simulink model "state_space"  (R2020b)
settings: Solver=VariableStepAuto  StartTime=0.0  StopTime=100  RelTol=1e-3
values from neighbouring files (symbols this model uses):
  A = [0 1 0 0 0; 0 0 0 0 0; 0 0 0 1 0; 0 0 0 0 1; 0 0 0 0 0]    [Kalman_vel_est.m]    (also in continues_time_state_space.m = [0 1 0 0; 0 0 0 0; 0 0 0 omega; 0 0 -omega 0])
  acc = test.data(:,28)    [acc_analysis.m]    (also in continues_time_state_space.m = 0)
  H = 100    [continues_time_state_space.m]
libraries: sharedTrackingLibrary x9, simulink x1
settings Model: Creator=Bruger  LastModifiedBy=Bruger

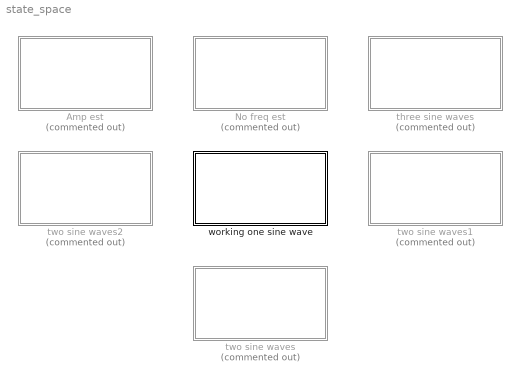
== system state_space ==
  Amp est : Subsystem  Commented=on
  No freq est : Subsystem  Commented=on
  three sine waves : Subsystem  Commented=on
  two sine waves : Subsystem  Commented=on
  two sine waves1 : Subsystem  Commented=on
  two sine waves2 : Subsystem  Commented=on
  working one sine wave : Subsystem

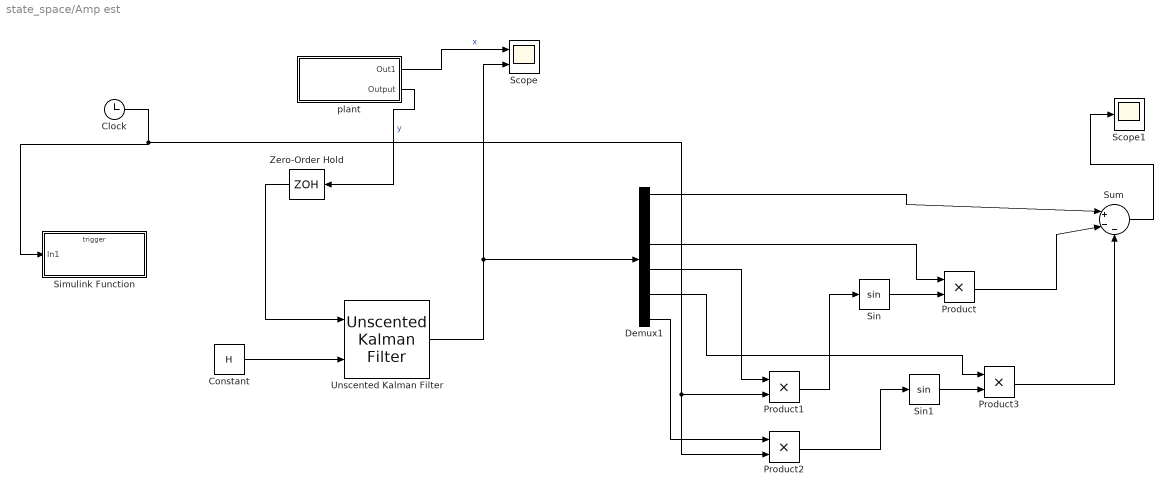
== system state_space/Amp est ==
  Clock : Clock
  Constant : Constant  Value=H
  Demux1 : Demux  Outputs=6
  Product{,1..3} (4 alike) : Product
  Scope : Scope  NumInputPorts=2
  Scope1 : Scope
  Simulink Function : Subsystem  TreatAsAtomicUnit=on
  Sin : Trigonometry
  Sin1 : Trigonometry
  Sum : Sum  Inputs=|+--
  Unscented Kalman Filter : sharedTrackingLibrary/Unscented Kalman Filter  StateTransitionFcn=state_transfer  HasAdditiveProcessNoise=Additive  ProcessNoise=0.01  HasTimeVaryingProcessNoise=off  HasStateTransitionFcnExtraArgument=0  InitialState=[100 0 40 2 20 1]  InitialStateCovariance=0.1  Alpha=1e-3  Beta=2  Kappa=0  MeasurementFcn1=f  HasMeasurementEnablePort1=off  HasAdditiveMeasurementNoise1=Additive  MeasurementNoise1=0.01  HasTimeVaryingMeasurementNoise1=off  HasMeasurementFcnExtraArgument1=0  MeasurementFcn2=measure_alt  HasMeasurementEnablePort2=off  HasAdditiveMeasurementNoise2=Additive  MeasurementNoise2=0.01  HasTimeVaryingMeasurementNoise2=off  HasMeasurementFcnExtraArgument2=0  MeasurementFcn3=myMeasurementFcn  HasMeasurementEnablePort3=off  HasAdditiveMeasurementNoise3=Additive  MeasurementNoise3=1  HasTimeVaryingMeasurementNoise3=off  HasMeasurementFcnExtraArgument3=0  MeasurementFcn4=myMeasurementFcn  HasMeasurementEnablePort4=off  HasAdditiveMeasurementNoise4=Additive  MeasurementNoise4=1  HasTimeVaryingMeasurementNoise4=off  HasMeasurementFcnExtraArgument4=0  MeasurementFcn5=myMeasurementFcn  HasMeasurementEnablePort5=off  HasAdditiveMeasurementNoise5=Additive  MeasurementNoise5=1  HasTimeVaryingMeasurementNoise5=off  HasMeasurementFcnExtraArgument5=0  EnableMultirate=off  StateTransitionFcnSampleTime=1  MeasurementFcn1SampleTime=1  MeasurementFcn2SampleTime=1  MeasurementFcn3SampleTime=1  MeasurementFcn4SampleTime=1  MeasurementFcn5SampleTime=1  UseCurrentEstimator=on  OutputStateCovariance=off  DataType=double  SampleTime=0.1  NumberOfMeasurements=2
      settings: SourceProductBaseCode=CT,DR,TF,ID,LP,NV,AR,RO,RR,UV,VE
  Zero-Order Hold : ZeroOrderHold  SampleTime=0.1
  plant : Subsystem
  wires:
  Zero-Order Hold/1 -> Unscented Kalman Filter/1
  plant/2(Output) -> Zero-Order Hold/1  "y"
  plant/1(Out1) -> Scope/1  "x"
  Constant/1 -> Unscented Kalman Filter/2
  Demux1/5 -> Product3/1
  Demux1/1 -> Sum/1
  Product3/1 -> Sum/3
  Demux1/3 -> Product/1
  Demux1/4 -> Product1/1
  Clock/1 -> Product2/2, Product1/2, Simulink Function/1(In1)
  Sin1/1 -> Product3/2
  Demux1/6 -> Product2/1
  Unscented Kalman Filter/1 -> Scope/2, Demux1/1
  Product/1 -> Sum/2
  Sin/1 -> Product/2
  Product2/1 -> Sin1/1
  Product1/1 -> Sin/1
  Sum/1 -> Scope1/1

== system state_space/No freq est ==
  Constant : Constant  Value=H
  Scope : Scope  NumInputPorts=2
  Scope1 : Scope
  Unscented Kalman Filter : sharedTrackingLibrary/Unscented Kalman Filter  StateTransitionFcn=state_transfer  HasAdditiveProcessNoise=Additive  ProcessNoise=1  HasTimeVaryingProcessNoise=off  HasStateTransitionFcnExtraArgument=0  InitialState=[100 0 0 10]  InitialStateCovariance=1  Alpha=1e-3  Beta=2  Kappa=0  MeasurementFcn1=measurement_func  HasMeasurementEnablePort1=off  HasAdditiveMeasurementNoise1=Additive  MeasurementNoise1=1  HasTimeVaryingMeasurementNoise1=off  HasMeasurementFcnExtraArgument1=0  MeasurementFcn2=measure_alt  HasMeasurementEnablePort2=off  HasAdditiveMeasurementNoise2=Additive  MeasurementNoise2=1  HasTimeVaryingMeasurementNoise2=off  HasMeasurementFcnExtraArgument2=0  MeasurementFcn3=myMeasurementFcn  HasMeasurementEnablePort3=off  HasAdditiveMeasurementNoise3=Additive  MeasurementNoise3=1  HasTimeVaryingMeasurementNoise3=off  HasMeasurementFcnExtraArgument3=0  MeasurementFcn4=myMeasurementFcn  HasMeasurementEnablePort4=off  HasAdditiveMeasurementNoise4=Additive  MeasurementNoise4=1  HasTimeVaryingMeasurementNoise4=off  HasMeasurementFcnExtraArgument4=0  MeasurementFcn5=myMeasurementFcn  HasMeasurementEnablePort5=off  HasAdditiveMeasurementNoise5=Additive  MeasurementNoise5=1  HasTimeVaryingMeasurementNoise5=off  HasMeasurementFcnExtraArgument5=0  EnableMultirate=off  StateTransitionFcnSampleTime=1  MeasurementFcn1SampleTime=1  MeasurementFcn2SampleTime=1  MeasurementFcn3SampleTime=1  MeasurementFcn4SampleTime=1  MeasurementFcn5SampleTime=1  UseCurrentEstimator=on  OutputStateCovariance=off  DataType=double  SampleTime=0.1  NumberOfMeasurements=2
      settings: SourceProductBaseCode=CT,DR,TF,ID,LP,NV,AR,RO,RR,UV,VE
  Zero-Order Hold : ZeroOrderHold  SampleTime=0.1
  plant : Subsystem
  wires:
  Zero-Order Hold/1 -> Unscented Kalman Filter/1
  plant/2(Output) -> Zero-Order Hold/1  "y"
  Unscented Kalman Filter/1 -> Scope/2
  plant/1(Out1) -> Scope/1  "x"
  Constant/1 -> Unscented Kalman Filter/2

== system state_space/three sine waves ==
  Constant : Constant  Value=H
  Demux : Demux  Outputs=11
  Demux1 : Demux  Outputs=8
  Scope : Scope  NumInputPorts=2
  Scope1 : Scope  NumInputPorts=6
  Scope2 : Scope  NumInputPorts=3
  Unscented Kalman Filter : sharedTrackingLibrary/Unscented Kalman Filter  StateTransitionFcn=state_transfer  HasAdditiveProcessNoise=Additive  ProcessNoise=1e-10  HasTimeVaryingProcessNoise=off  HasStateTransitionFcnExtraArgument=0  InitialState=[50 0 0 10 1 0 5 4 0 20 2]  InitialStateCovariance=1e-10  Alpha=1e-3  Beta=1  Kappa=0  MeasurementFcn1=measurement_func  HasMeasurementEnablePort1=off  HasAdditiveMeasurementNoise1=Additive  MeasurementNoise1=1e-10  HasTimeVaryingMeasurementNoise1=off  HasMeasurementFcnExtraArgument1=0  MeasurementFcn2=measure_alt  HasMeasurementEnablePort2=off  HasAdditiveMeasurementNoise2=Additive  MeasurementNoise2=1e-10  HasTimeVaryingMeasurementNoise2=off  HasMeasurementFcnExtraArgument2=0  MeasurementFcn3=myMeasurementFcn  HasMeasurementEnablePort3=off  HasAdditiveMeasurementNoise3=Additive  MeasurementNoise3=1  HasTimeVaryingMeasurementNoise3=off  HasMeasurementFcnExtraArgument3=0  MeasurementFcn4=myMeasurementFcn  HasMeasurementEnablePort4=off  HasAdditiveMeasurementNoise4=Additive  MeasurementNoise4=1  HasTimeVaryingMeasurementNoise4=off  HasMeasurementFcnExtraArgument4=0  MeasurementFcn5=myMeasurementFcn  HasMeasurementEnablePort5=off  HasAdditiveMeasurementNoise5=Additive  MeasurementNoise5=1  HasTimeVaryingMeasurementNoise5=off  HasMeasurementFcnExtraArgument5=0  EnableMultirate=off  StateTransitionFcnSampleTime=1  MeasurementFcn1SampleTime=1  MeasurementFcn2SampleTime=1  MeasurementFcn3SampleTime=1  MeasurementFcn4SampleTime=1  MeasurementFcn5SampleTime=1  UseCurrentEstimator=on  OutputStateCovariance=off  DataType=double  SampleTime=0.1  NumberOfMeasurements=2
      settings: SourceProductBaseCode=CT,DR,TF,ID,LP,NV,AR,RO,RR,UV,VE
  Zero-Order Hold : ZeroOrderHold  SampleTime=0.1
  plant : Subsystem
  wires:
  Zero-Order Hold/1 -> Unscented Kalman Filter/1
  plant/2(Output) -> Zero-Order Hold/1  "y"
  Unscented Kalman Filter/1 -> Scope/2, Demux/1
  plant/1(Out1) -> Demux1/1, Scope/1  "x"
  Constant/1 -> Unscented Kalman Filter/2
  Demux/6 -> Scope1/5  "sine_est2"
  Demux1/5 -> Scope1/1  "sine_gt2"
  Demux/3 -> Scope1/4  "sine_est1"
  Demux1/3 -> Scope1/2  "sine_gt1"
  Demux/8 -> Scope2/3  "freq"
  Demux/5 -> Scope2/2
  Demux/11 -> Scope2/1
  Demux1/7 -> Scope1/3  "sine_gt3"
  Demux/9 -> Scope1/6  "sine_est3"

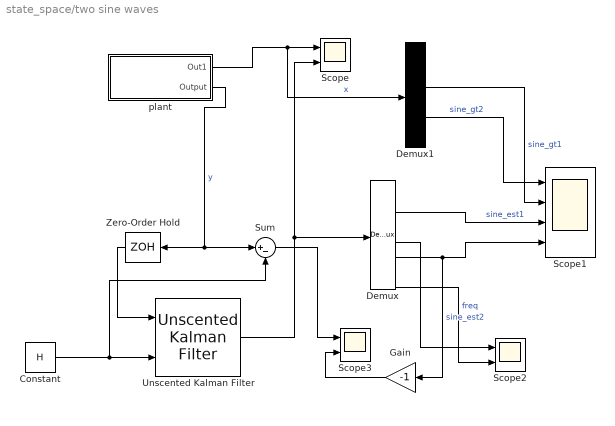
== system state_space/two sine waves ==
  Constant : Constant  Value=H
  Demux : Demux  Outputs=8
  Demux1 : Demux  Outputs=6
  Gain : Gain  Gain=-1
  Scope : Scope  NumInputPorts=2
  Scope1 : Scope  NumInputPorts=4
  Scope2 : Scope  NumInputPorts=2
  Scope3 : Scope  NumInputPorts=2
  Sum : Sum  Inputs=|+-
  Unscented Kalman Filter : sharedTrackingLibrary/Unscented Kalman Filter  StateTransitionFcn=state_transfer  HasAdditiveProcessNoise=Additive  ProcessNoise=0.1  HasTimeVaryingProcessNoise=off  HasStateTransitionFcnExtraArgument=0  InitialState=[100 0 0 40 2.5 0 20 1.5]  InitialStateCovariance=1  Alpha=1e-3  Beta=2  Kappa=0  MeasurementFcn1=measurement_func  HasMeasurementEnablePort1=off  HasAdditiveMeasurementNoise1=Additive  MeasurementNoise1=0.1  HasTimeVaryingMeasurementNoise1=off  HasMeasurementFcnExtraArgument1=0  MeasurementFcn2=measure_alt  HasMeasurementEnablePort2=off  HasAdditiveMeasurementNoise2=Additive  MeasurementNoise2=0.1  HasTimeVaryingMeasurementNoise2=off  HasMeasurementFcnExtraArgument2=0  MeasurementFcn3=myMeasurementFcn  HasMeasurementEnablePort3=off  HasAdditiveMeasurementNoise3=Additive  MeasurementNoise3=1  HasTimeVaryingMeasurementNoise3=off  HasMeasurementFcnExtraArgument3=0  MeasurementFcn4=myMeasurementFcn  HasMeasurementEnablePort4=off  HasAdditiveMeasurementNoise4=Additive  MeasurementNoise4=1  HasTimeVaryingMeasurementNoise4=off  HasMeasurementFcnExtraArgument4=0  MeasurementFcn5=myMeasurementFcn  HasMeasurementEnablePort5=off  HasAdditiveMeasurementNoise5=Additive  MeasurementNoise5=1  HasTimeVaryingMeasurementNoise5=off  HasMeasurementFcnExtraArgument5=0  EnableMultirate=off  StateTransitionFcnSampleTime=1  MeasurementFcn1SampleTime=1  MeasurementFcn2SampleTime=1  MeasurementFcn3SampleTime=1  MeasurementFcn4SampleTime=1  MeasurementFcn5SampleTime=1  UseCurrentEstimator=on  OutputStateCovariance=off  DataType=double  SampleTime=0.1  NumberOfMeasurements=2
      settings: SourceProductBaseCode=CT,DR,TF,ID,LP,NV,AR,RO,RR,UV,VE
  Zero-Order Hold : ZeroOrderHold  SampleTime=0.1
  plant : Subsystem
  wires:
  Zero-Order Hold/1 -> Unscented Kalman Filter/1
  plant/2(Output) -> Zero-Order Hold/1, Sum/1  "y"
  Unscented Kalman Filter/1 -> Scope/2, Demux/1
  plant/1(Out1) -> Demux1/1, Scope/1  "x"
  Constant/1 -> Sum/2, Unscented Kalman Filter/2
  Demux/6 -> Gain/1, Scope1/4  "sine_est2"
  Demux1/5 -> Scope1/1  "sine_gt2"
  Demux/3 -> Scope1/3  "sine_est1"
  Demux1/3 -> Scope1/2  "sine_gt1"
  Demux/8 -> Scope2/2  "freq"
  Demux/5 -> Scope2/1
  Sum/1 -> Scope3/1
  Gain/1 -> Scope3/2

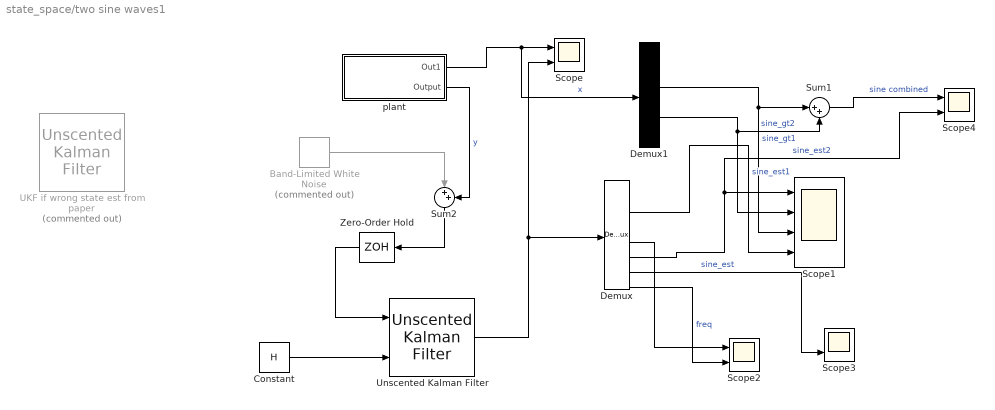
== system state_space/two sine waves1 ==
  Band-Limited White Noise : simulink/Sources/Band-Limited White Noise  Commented=on  Cov=[0.1]  Ts=0.05  seed=[23341]
  Constant : Constant  Value=H
  Demux : Demux  Outputs=8
  Demux1 : Demux  Outputs=6
  Scope{,2..4} (4 alike) : Scope  NumInputPorts=2
  Scope1 : Scope  NumInputPorts=4
  Sum1 : Sum  Inputs=|++
  Sum2 : Sum  Inputs=|++
  UKF if wrong state est from paper : sharedTrackingLibrary/Unscented Kalman Filter  Commented=on  StateTransitionFcn=state_transfer  HasAdditiveProcessNoise=Additive  ProcessNoise=0.01  HasTimeVaryingProcessNoise=off  HasStateTransitionFcnExtraArgument=0  InitialState=[100 0 0 20 0.5 0 40 1]  InitialStateCovariance=0.01  Alpha=1e-3  Beta=2  Kappa=0  MeasurementFcn1=measurement_func  HasMeasurementEnablePort1=off  HasAdditiveMeasurementNoise1=Additive  MeasurementNoise1=0.04  HasTimeVaryingMeasurementNoise1=off  HasMeasurementFcnExtraArgument1=0  MeasurementFcn2=measure_alt  HasMeasurementEnablePort2=off  HasAdditiveMeasurementNoise2=Additive  MeasurementNoise2=0.1  HasTimeVaryingMeasurementNoise2=off  HasMeasurementFcnExtraArgument2=0  MeasurementFcn3=myMeasurementFcn  HasMeasurementEnablePort3=off  HasAdditiveMeasurementNoise3=Additive  MeasurementNoise3=1  HasTimeVaryingMeasurementNoise3=off  HasMeasurementFcnExtraArgument3=0  MeasurementFcn4=myMeasurementFcn  HasMeasurementEnablePort4=off  HasAdditiveMeasurementNoise4=Additive  MeasurementNoise4=1  HasTimeVaryingMeasurementNoise4=off  HasMeasurementFcnExtraArgument4=0  MeasurementFcn5=myMeasurementFcn  HasMeasurementEnablePort5=off  HasAdditiveMeasurementNoise5=Additive  MeasurementNoise5=1  HasTimeVaryingMeasurementNoise5=off  HasMeasurementFcnExtraArgument5=0  EnableMultirate=off  StateTransitionFcnSampleTime=1  MeasurementFcn1SampleTime=1  MeasurementFcn2SampleTime=1  MeasurementFcn3SampleTime=1  MeasurementFcn4SampleTime=1  MeasurementFcn5SampleTime=1  UseCurrentEstimator=on  OutputStateCovariance=off  DataType=double  SampleTime=0.05  NumberOfMeasurements=2
      settings: SourceProductBaseCode=CT,DR,TF,ID,LP,NV,AR,RO,RR,UV,VE
  Unscented Kalman Filter : sharedTrackingLibrary/Unscented Kalman Filter  StateTransitionFcn=state_transfer  HasAdditiveProcessNoise=Additive  ProcessNoise=0.1  HasTimeVaryingProcessNoise=off  HasStateTransitionFcnExtraArgument=0  InitialState=[100 0 0 20 0.5 0 40 1]  InitialStateCovariance=0.1  Alpha=1e-3  Beta=2  Kappa=0  MeasurementFcn1=measurement_func  HasMeasurementEnablePort1=off  HasAdditiveMeasurementNoise1=Additive  MeasurementNoise1=0.1  HasTimeVaryingMeasurementNoise1=off  HasMeasurementFcnExtraArgument1=0  MeasurementFcn2=measure_alt  HasMeasurementEnablePort2=off  HasAdditiveMeasurementNoise2=Additive  MeasurementNoise2=0.1  HasTimeVaryingMeasurementNoise2=off  HasMeasurementFcnExtraArgument2=0  MeasurementFcn3=myMeasurementFcn  HasMeasurementEnablePort3=off  HasAdditiveMeasurementNoise3=Additive  MeasurementNoise3=1  HasTimeVaryingMeasurementNoise3=off  HasMeasurementFcnExtraArgument3=0  MeasurementFcn4=myMeasurementFcn  HasMeasurementEnablePort4=off  HasAdditiveMeasurementNoise4=Additive  MeasurementNoise4=1  HasTimeVaryingMeasurementNoise4=off  HasMeasurementFcnExtraArgument4=0  MeasurementFcn5=myMeasurementFcn  HasMeasurementEnablePort5=off  HasAdditiveMeasurementNoise5=Additive  MeasurementNoise5=1  HasTimeVaryingMeasurementNoise5=off  HasMeasurementFcnExtraArgument5=0  EnableMultirate=off  StateTransitionFcnSampleTime=1  MeasurementFcn1SampleTime=1  MeasurementFcn2SampleTime=1  MeasurementFcn3SampleTime=1  MeasurementFcn4SampleTime=1  MeasurementFcn5SampleTime=1  UseCurrentEstimator=on  OutputStateCovariance=off  DataType=double  SampleTime=0.02  NumberOfMeasurements=2
      settings: SourceProductBaseCode=CT,DR,TF,ID,LP,NV,AR,RO,RR,UV,VE
  Zero-Order Hold : ZeroOrderHold  SampleTime=0.02
  plant : Subsystem
  wires:
  Zero-Order Hold/1 -> Unscented Kalman Filter/1
  Unscented Kalman Filter/1 -> Scope/2, Demux/1
  plant/1(Out1) -> Demux1/1, Scope/1  "x"
  Constant/1 -> Unscented Kalman Filter/2
  Demux/6 -> Scope4/2, Scope1/1  "sine_est2"
  Demux1/5 -> Sum1/2, Scope1/2  "sine_gt2"
  Demux/3 -> Scope1/4  "sine_est1"
  Demux1/3 -> Sum1/1, Scope1/3  "sine_gt1"
  Demux/8 -> Scope2/2  "freq"
  Demux/5 -> Scope2/1
  Sum1/1 -> Scope4/1  "sine combined"
  Band-Limited White Noise/1 -> Sum2/1
  plant/2(Output) -> Sum2/2  "y"
  Sum2/1 -> Zero-Order Hold/1
  Demux/7 -> Scope3/2  "sine_est"

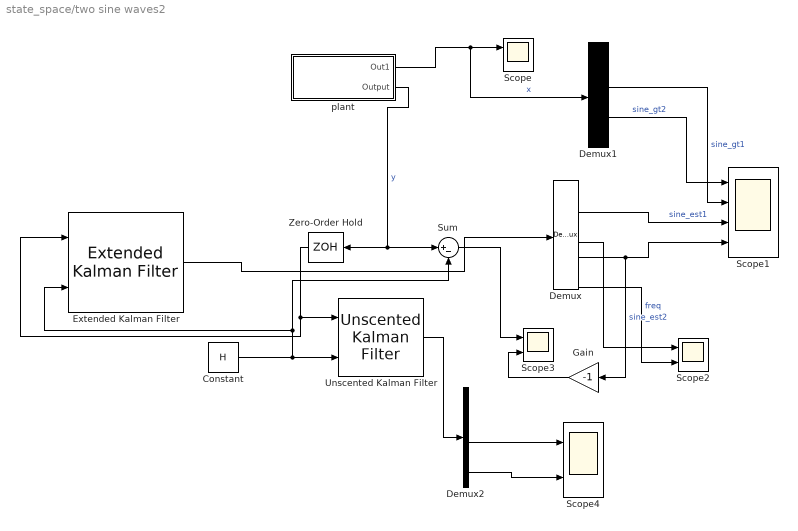
== system state_space/two sine waves2 ==
  Constant : Constant  Value=H
  Demux : Demux  Outputs=8
  Demux1 : Demux  Outputs=6
  Demux2 : Demux  Outputs=8
  Extended Kalman Filter : sharedTrackingLibrary/Extended Kalman Filter  StateTransitionFcn=state_transfer  HasStateTransitionJacobianFcn=off  HasAdditiveProcessNoise=Additive  ProcessNoise=0.1  HasTimeVaryingProcessNoise=off  HasStateTransitionFcnExtraArgument=0  InitialState=[100 0 0 40 2.5 0 20 1.5]  InitialStateCovariance=0.1  MeasurementFcn1=measurement_func  HasMeasurementJacobianFcn1=off  HasMeasurementEnablePort1=off  HasAdditiveMeasurementNoise1=Additive  MeasurementNoise1=0.1  HasTimeVaryingMeasurementNoise1=off  HasMeasurementFcnExtraArgument1=0  MeasurementFcn2=measure_alt  HasMeasurementJacobianFcn2=off  HasMeasurementEnablePort2=off  HasAdditiveMeasurementNoise2=Additive  MeasurementNoise2=0.1  HasTimeVaryingMeasurementNoise2=off  HasMeasurementFcnExtraArgument2=0  MeasurementFcn3=myMeasurementFcn  HasMeasurementJacobianFcn3=off  HasMeasurementEnablePort3=off  HasAdditiveMeasurementNoise3=Additive  MeasurementNoise3=1  HasTimeVaryingMeasurementNoise3=off  HasMeasurementFcnExtraArgument3=0  MeasurementFcn4=myMeasurementFcn  HasMeasurementJacobianFcn4=off  HasMeasurementEnablePort4=off  HasAdditiveMeasurementNoise4=Additive  MeasurementNoise4=1  HasTimeVaryingMeasurementNoise4=off  HasMeasurementFcnExtraArgument4=0  MeasurementFcn5=myMeasurementFcn  HasMeasurementJacobianFcn5=off  HasMeasurementEnablePort5=off  HasAdditiveMeasurementNoise5=Additive  MeasurementNoise5=1  HasTimeVaryingMeasurementNoise5=off  HasMeasurementFcnExtraArgument5=0  EnableMultirate=off  StateTransitionFcnSampleTime=1  MeasurementFcn1SampleTime=1  MeasurementFcn2SampleTime=1  MeasurementFcn3SampleTime=1  MeasurementFcn4SampleTime=1  MeasurementFcn5SampleTime=1  UseCurrentEstimator=on  OutputStateCovariance=off  DataType=double  SampleTime=0.1  NumberOfMeasurements=2
      settings: SourceProductBaseCode=CT,DR,TF,ID,LP,NV,AR,RO,RR,UV,VE
  Gain : Gain  Gain=-1
  Scope{,2..4} (4 alike) : Scope  NumInputPorts=2
  Scope1 : Scope  NumInputPorts=4
  Sum : Sum  Inputs=|+-
  Unscented Kalman Filter : sharedTrackingLibrary/Unscented Kalman Filter  StateTransitionFcn=state_transfer  HasAdditiveProcessNoise=Additive  ProcessNoise=0.01  HasTimeVaryingProcessNoise=off  HasStateTransitionFcnExtraArgument=0  InitialState=[100 0 0 40 2.5 0 20 1.5]  InitialStateCovariance=0.1  Alpha=1e-3  Beta=2  Kappa=0  MeasurementFcn1=measurement_func  HasMeasurementEnablePort1=off  HasAdditiveMeasurementNoise1=Additive  MeasurementNoise1=0.1  HasTimeVaryingMeasurementNoise1=off  HasMeasurementFcnExtraArgument1=0  MeasurementFcn2=measure_alt  HasMeasurementEnablePort2=off  HasAdditiveMeasurementNoise2=Additive  MeasurementNoise2=0.1  HasTimeVaryingMeasurementNoise2=off  HasMeasurementFcnExtraArgument2=0  MeasurementFcn3=myMeasurementFcn  HasMeasurementEnablePort3=off  HasAdditiveMeasurementNoise3=Additive  MeasurementNoise3=1  HasTimeVaryingMeasurementNoise3=off  HasMeasurementFcnExtraArgument3=0  MeasurementFcn4=myMeasurementFcn  HasMeasurementEnablePort4=off  HasAdditiveMeasurementNoise4=Additive  MeasurementNoise4=1  HasTimeVaryingMeasurementNoise4=off  HasMeasurementFcnExtraArgument4=0  MeasurementFcn5=myMeasurementFcn  HasMeasurementEnablePort5=off  HasAdditiveMeasurementNoise5=Additive  MeasurementNoise5=1  HasTimeVaryingMeasurementNoise5=off  HasMeasurementFcnExtraArgument5=0  EnableMultirate=off  StateTransitionFcnSampleTime=1  MeasurementFcn1SampleTime=1  MeasurementFcn2SampleTime=1  MeasurementFcn3SampleTime=1  MeasurementFcn4SampleTime=1  MeasurementFcn5SampleTime=1  UseCurrentEstimator=on  OutputStateCovariance=off  DataType=double  SampleTime=0.1  NumberOfMeasurements=2
      settings: SourceProductBaseCode=CT,DR,TF,ID,LP,NV,AR,RO,RR,UV,VE
  Zero-Order Hold : ZeroOrderHold  SampleTime=0.1
  plant : Subsystem
  wires:
  Zero-Order Hold/1 -> Unscented Kalman Filter/1, Extended Kalman Filter/1
  plant/2(Output) -> Zero-Order Hold/1, Sum/1  "y"
  plant/1(Out1) -> Demux1/1, Scope/1  "x"
  Constant/1 -> Extended Kalman Filter/2, Sum/2, Unscented Kalman Filter/2
  Demux/6 -> Gain/1, Scope1/4  "sine_est2"
  Demux1/5 -> Scope1/1  "sine_gt2"
  Demux/3 -> Scope1/3  "sine_est1"
  Demux1/3 -> Scope1/2  "sine_gt1"
  Demux/8 -> Scope2/2  "freq"
  Demux/5 -> Scope2/1
  Sum/1 -> Scope3/1
  Gain/1 -> Scope3/2
  Extended Kalman Filter/1 -> Demux/1
  Unscented Kalman Filter/1 -> Demux2/1
  Demux2/8 -> Scope4/2
  Demux2/5 -> Scope4/1

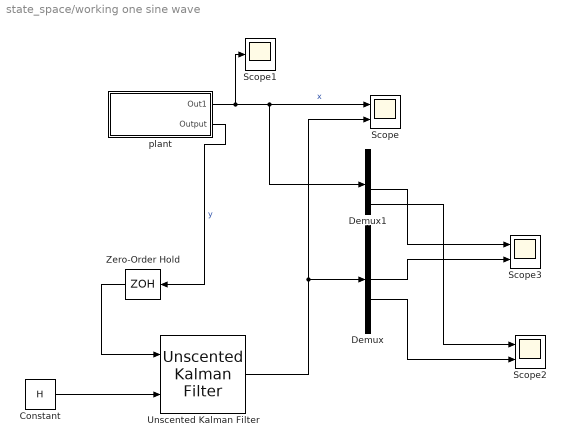
== system state_space/working one sine wave ==
  Constant : Constant  Value=H
  Demux : Demux  Outputs=5
  Demux1 : Demux
  Scope : Scope  NumInputPorts=2
  Scope1 : Scope
  Scope2 : Scope  NumInputPorts=2
  Scope3 : Scope  NumInputPorts=2
  Unscented Kalman Filter : sharedTrackingLibrary/Unscented Kalman Filter  StateTransitionFcn=state_transfer  HasAdditiveProcessNoise=Additive  ProcessNoise=0.1  HasTimeVaryingProcessNoise=off  HasStateTransitionFcnExtraArgument=0  InitialState=[100 0 0 10 1]  InitialStateCovariance=0.1  Alpha=1e-3  Beta=2  Kappa=0  MeasurementFcn1=measurement_func  HasMeasurementEnablePort1=off  HasAdditiveMeasurementNoise1=Additive  MeasurementNoise1=0.1  HasTimeVaryingMeasurementNoise1=off  HasMeasurementFcnExtraArgument1=0  MeasurementFcn2=measure_alt  HasMeasurementEnablePort2=off  HasAdditiveMeasurementNoise2=Additive  MeasurementNoise2=0.1  HasTimeVaryingMeasurementNoise2=off  HasMeasurementFcnExtraArgument2=0  MeasurementFcn3=myMeasurementFcn  HasMeasurementEnablePort3=off  HasAdditiveMeasurementNoise3=Additive  MeasurementNoise3=1  HasTimeVaryingMeasurementNoise3=off  HasMeasurementFcnExtraArgument3=0  MeasurementFcn4=myMeasurementFcn  HasMeasurementEnablePort4=off  HasAdditiveMeasurementNoise4=Additive  MeasurementNoise4=1  HasTimeVaryingMeasurementNoise4=off  HasMeasurementFcnExtraArgument4=0  MeasurementFcn5=myMeasurementFcn  HasMeasurementEnablePort5=off  HasAdditiveMeasurementNoise5=Additive  MeasurementNoise5=1  HasTimeVaryingMeasurementNoise5=off  HasMeasurementFcnExtraArgument5=0  EnableMultirate=off  StateTransitionFcnSampleTime=1  MeasurementFcn1SampleTime=1  MeasurementFcn2SampleTime=1  MeasurementFcn3SampleTime=1  MeasurementFcn4SampleTime=1  MeasurementFcn5SampleTime=1  UseCurrentEstimator=on  OutputStateCovariance=off  DataType=double  SampleTime=0.1  NumberOfMeasurements=2
      settings: SourceProductBaseCode=CT,DR,TF,ID,LP,NV,AR,RO,RR,UV,VE
  Zero-Order Hold : ZeroOrderHold  SampleTime=0.1
  plant : Subsystem
  wires:
  Zero-Order Hold/1 -> Unscented Kalman Filter/1
  plant/2(Output) -> Zero-Order Hold/1  "y"
  plant/1(Out1) -> Demux1/1, Scope/1, Scope1/1  "x"
  Constant/1 -> Unscented Kalman Filter/2
  Unscented Kalman Filter/1 -> Demux/1, Scope/2
  Demux1/4 -> Scope2/1
  Demux/4 -> Scope2/2
  Demux1/3 -> Scope3/1
  Demux/3 -> Scope3/2

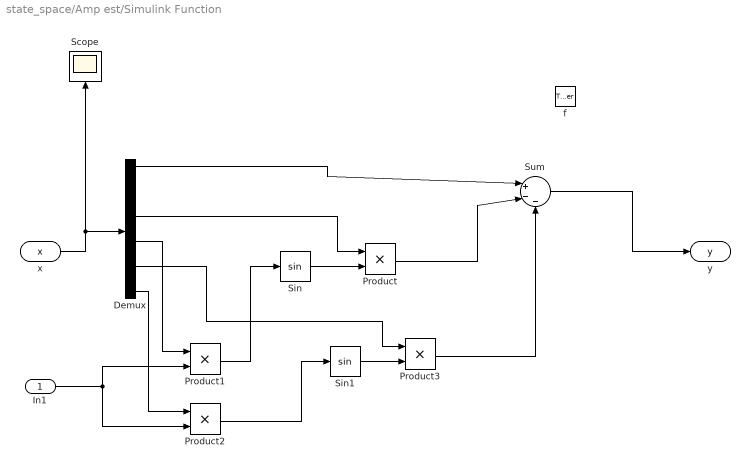
== system state_space/Amp est/Simulink Function ==
  In1 : Inport
  f : TriggerPort  TriggerType=function-call  IsSimulinkFunction=on  FunctionName=f  FunctionVisibility=scoped  VariantControl=(inherit)
  Demux : Demux  Outputs=6
  Product{,1..3} (4 alike) : Product
  Scope : Scope
  Sin : Trigonometry
  Sin1 : Trigonometry
  Sum : Sum  Inputs=|+--
  x : ArgIn  DisableCoverage=on  PortDimensions=6  ArgumentName=x
  y : ArgOut  DisableCoverage=on  ArgumentName=y
  wires:
  x/1 -> Demux/1, Scope/1
  Demux/1 -> Sum/1
  Sin/1 -> Product/2
  In1/1 -> Product2/2, Product1/2
  Product1/1 -> Sin/1
  Product/1 -> Sum/2
  Product2/1 -> Sin1/1
  Sin1/1 -> Product3/2
  Product3/1 -> Sum/3
  Sum/1 -> y/1
  Demux/3 -> Product/1
  Demux/4 -> Product1/1
  Demux/5 -> Product3/1
  Demux/6 -> Product2/1

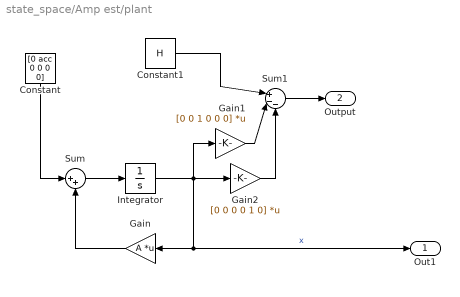
== system state_space/Amp est/plant ==
  Constant : Constant  Value=[0 acc 0 0 0 0]
  Constant1 : Constant  Value=H
  Gain : Gain  Gain=A  Multiplication=Matrix(K*u) (u vector)
  Gain1 : Gain  Gain=[0 0 1 0 0 0]  Multiplication=Matrix(K*u) (u vector)
  Gain2 : Gain  Gain=[0 0 0 0 1 0]  Multiplication=Matrix(K*u) (u vector)
  Integrator : Integrator  InitialCondition=[H 0 0 40 0 20]
  Sum : Sum  Inputs=|++
  Sum1 : Sum  Inputs=|+--
  Out1 : Outport
  Output : Outport  Port=2
  wires:
  Integrator/1 -> Gain2/1, Gain/1, Out1/1, Gain1/1  "x"
  Gain/1 -> Sum/2
  Constant/1 -> Sum/1
  Sum/1 -> Integrator/1
  Sum1/1 -> Output/1
  Constant1/1 -> Sum1/1
  Gain1/1 -> Sum1/2
  Gain2/1 -> Sum1/3

== system state_space/No freq est/plant ==
  Constant : Constant  Value=[0 acc 0 0]
  Constant1 : Constant  Value=H
  Gain : Gain  Gain=A  Multiplication=Matrix(K*u) (u vector)
  Gain1 : Gain  Gain=[0 0 1 0]  Multiplication=Matrix(K*u) (u vector)
  Integrator : Integrator  InitialCondition=[H 0 0 10]
  Sum : Sum  Inputs=|++
  Sum1 : Sum  Inputs=|+-
  Out1 : Outport
  Output : Outport  Port=2
  wires:
  Integrator/1 -> Gain1/1, Gain/1, Out1/1  "x"
  Gain/1 -> Sum/2
  Constant/1 -> Sum/1
  Sum/1 -> Integrator/1
  Sum1/1 -> Output/1
  Constant1/1 -> Sum1/1
  Gain1/1 -> Sum1/2

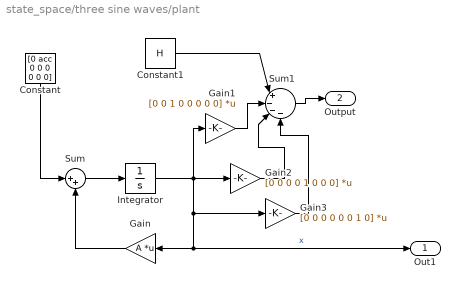
== system state_space/three sine waves/plant ==
  Constant : Constant  Value=[0 acc 0 0 0 0 0 0]
  Constant1 : Constant  Value=H
  Gain : Gain  Gain=A  Multiplication=Matrix(K*u) (u vector)
  Gain1 : Gain  Gain=[0 0 1 0 0 0 0 0]  Multiplication=Matrix(K*u) (u vector)
  Gain2 : Gain  Gain=[0 0 0 0 1 0 0 0]  Multiplication=Matrix(K*u) (u vector)
  Gain3 : Gain  Gain=[0 0 0 0 0 0 1 0]  Multiplication=Matrix(K*u) (u vector)
  Integrator : Integrator  InitialCondition=[H 0 0 10 0 5 0 20]
  Sum : Sum  Inputs=|++
  Sum1 : Sum  Inputs=|+---
  Out1 : Outport
  Output : Outport  Port=2
  wires:
  Integrator/1 -> Gain3/1, Gain/1, Out1/1, Gain2/1, Gain1/1  "x"
  Gain/1 -> Sum/2
  Constant/1 -> Sum/1
  Sum/1 -> Integrator/1
  Sum1/1 -> Output/1
  Constant1/1 -> Sum1/1
  Gain1/1 -> Sum1/2
  Gain2/1 -> Sum1/3
  Gain3/1 -> Sum1/4

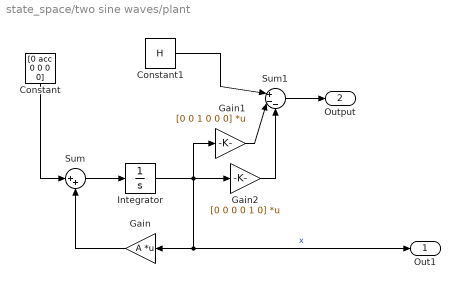
== system state_space/two sine waves/plant ==
  Constant : Constant  Value=[0 acc 0 0 0 0]
  Constant1 : Constant  Value=H
  Gain : Gain  Gain=A  Multiplication=Matrix(K*u) (u vector)
  Gain1 : Gain  Gain=[0 0 1 0 0 0]  Multiplication=Matrix(K*u) (u vector)
  Gain2 : Gain  Gain=[0 0 0 0 1 0]  Multiplication=Matrix(K*u) (u vector)
  Integrator : Integrator  InitialCondition=[H 0 0 40 0 20]
  Sum : Sum  Inputs=|++
  Sum1 : Sum  Inputs=|+--
  Out1 : Outport
  Output : Outport  Port=2
  wires:
  Integrator/1 -> Gain2/1, Gain/1, Out1/1, Gain1/1  "x"
  Gain/1 -> Sum/2
  Constant/1 -> Sum/1
  Sum/1 -> Integrator/1
  Sum1/1 -> Output/1
  Constant1/1 -> Sum1/1
  Gain1/1 -> Sum1/2
  Gain2/1 -> Sum1/3

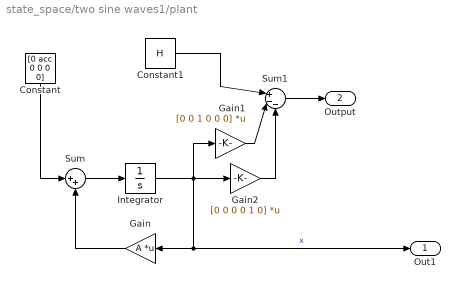
== system state_space/two sine waves1/plant ==
  Constant : Constant  Value=[0 acc 0 0 0 0]
  Constant1 : Constant  Value=H
  Gain : Gain  Gain=A  Multiplication=Matrix(K*u) (u vector)
  Gain1 : Gain  Gain=[0 0 1 0 0 0]  Multiplication=Matrix(K*u) (u vector)
  Gain2 : Gain  Gain=[0 0 0 0 1 0]  Multiplication=Matrix(K*u) (u vector)
  Integrator : Integrator  InitialCondition=[H 0 0 40 0 20]
  Sum : Sum  Inputs=|++
  Sum1 : Sum  Inputs=|+--
  Out1 : Outport
  Output : Outport  Port=2
  wires:
  Integrator/1 -> Gain2/1, Gain/1, Out1/1, Gain1/1  "x"
  Gain/1 -> Sum/2
  Constant/1 -> Sum/1
  Sum/1 -> Integrator/1
  Sum1/1 -> Output/1
  Constant1/1 -> Sum1/1
  Gain1/1 -> Sum1/2
  Gain2/1 -> Sum1/3

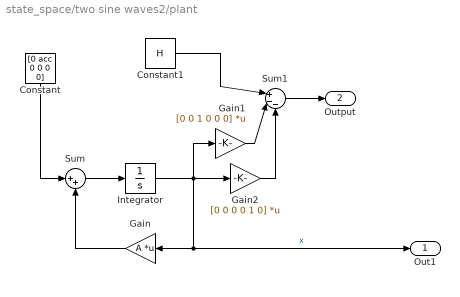
== system state_space/two sine waves2/plant ==
  Constant : Constant  Value=[0 acc 0 0 0 0]
  Constant1 : Constant  Value=H
  Gain : Gain  Gain=A  Multiplication=Matrix(K*u) (u vector)
  Gain1 : Gain  Gain=[0 0 1 0 0 0]  Multiplication=Matrix(K*u) (u vector)
  Gain2 : Gain  Gain=[0 0 0 0 1 0]  Multiplication=Matrix(K*u) (u vector)
  Integrator : Integrator  InitialCondition=[H 0 0 40 0 20]
  Sum : Sum  Inputs=|++
  Sum1 : Sum  Inputs=|+--
  Out1 : Outport
  Output : Outport  Port=2
  wires:
  Integrator/1 -> Gain2/1, Gain/1, Out1/1, Gain1/1  "x"
  Gain/1 -> Sum/2
  Constant/1 -> Sum/1
  Sum/1 -> Integrator/1
  Sum1/1 -> Output/1
  Constant1/1 -> Sum1/1
  Gain1/1 -> Sum1/2
  Gain2/1 -> Sum1/3

== system state_space/working one sine wave/plant ==
  Constant : Constant  Value=[0 acc 0 0]
  Constant1 : Constant  Value=H
  Gain : Gain  Gain=A  Multiplication=Matrix(K*u) (u vector)
  Gain1 : Gain  Gain=[0 0 1 0]  Multiplication=Matrix(K*u) (u vector)
  Integrator : Integrator  InitialCondition=[H 0 0 10]
  Scope : Scope
  Sum : Sum  Inputs=|++
  Sum1 : Sum  Inputs=|+-
  Out1 : Outport
  Output : Outport  Port=2
  wires:
  Integrator/1 -> Gain/1, Scope/1, Out1/1, Gain1/1  "x"
  Gain/1 -> Sum/2
  Constant/1 -> Sum/1
  Sum/1 -> Integrator/1
  Sum1/1 -> Output/1
  Constant1/1 -> Sum1/1
  Gain1/1 -> Sum1/2
